simulink library "rect_model"  (R2018a)
settings: Solver=VariableStepAuto  StartTime=0.0  StopTime=10.0  RelTol=1e-3
libraries: powerlib x9
settings Model: Creator=ASUS  LastModifiedBy=ASUS

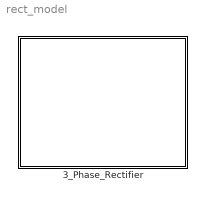
== system rect_model ==
  3_Phase_Rectifier : Subsystem

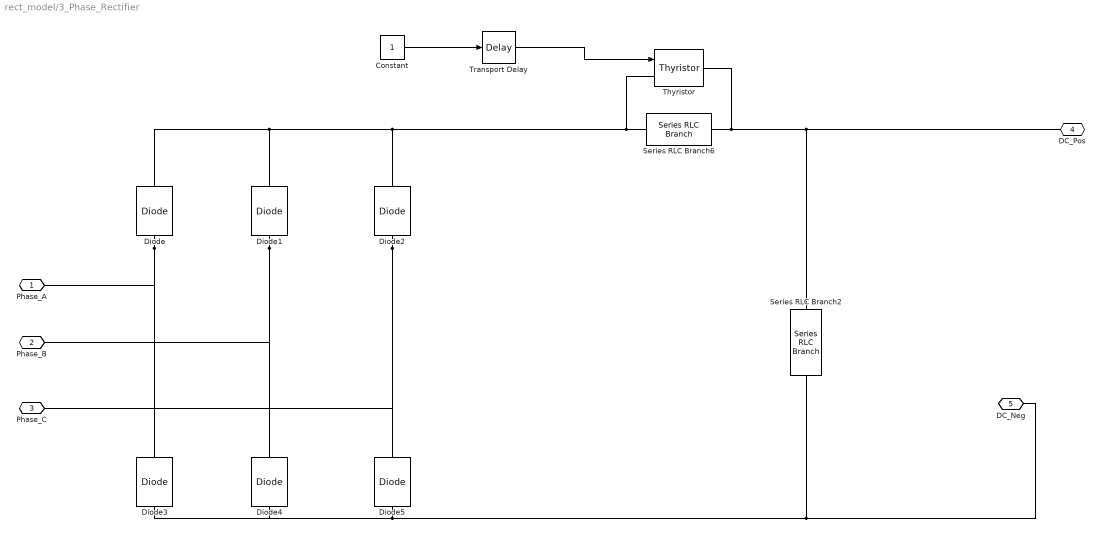
== system rect_model/3_Phase_Rectifier ==
  Constant : Constant
  Diode{,1..5} (6 alike) : powerlib/Power Electronics/Diode  Ron=0.001  Lon=0  Vf=0.8  IC=0  UseSnubber=0  Rs=500  Cs=250e-9  Measurements=off
  Series RLC Branch2 : powerlib/Elements/Series RLC Branch  LConnTagsString=__new0  RConnTagsString=__new0  BranchType=C  Resistance=72  Inductance=1e-3  SetiL0=off  InitialCurrent=0  Capacitance=2e-3  Setx0=off  InitialVoltage=0  Measurements=None
  Series RLC Branch6 : powerlib/Elements/Series RLC Branch  LConnTagsString=__new0  RConnTagsString=__new0  BranchType=R  Resistance=72  Inductance=1e-3  SetiL0=off  InitialCurrent=0  Capacitance=1e-6  Setx0=off  InitialVoltage=0  Measurements=None
  Thyristor : powerlib/Power Electronics/Thyristor  Ron=0.001  Lon=0  Vf=0.8  IC=0  Rs=500  Cs=250e-9  Measurements=off
  Transport Delay : TransportDelay  DelayTime=0.2
  Phase_A : PMIOPort  Side=Left
  Phase_B : PMIOPort  Port=2  Side=Left
  Phase_C : PMIOPort  Port=3  Side=Left
  DC_Pos : PMIOPort  Port=4  Side=Right
  DC_Neg : PMIOPort  Port=5  Side=Right
  wires:
  Transport Delay/1 -> Thyristor/1
  Constant/1 -> Transport Delay/1
  connections:
  Diode2/LConn1 -- Diode5/RConn1 -- Phase_C/RConn1
  Thyristor/LConn1 -- Series RLC Branch6/LConn1 -- Diode2/RConn1 -- Diode1/RConn1 -- Diode/RConn1
  Thyristor/RConn1 -- Series RLC Branch6/RConn1 -- Series RLC Branch2/LConn1 -- DC_Pos/RConn1
  Series RLC Branch2/RConn1 -- Diode3/LConn1 -- Diode4/LConn1 -- Diode5/LConn1 -- DC_Neg/RConn1
  Diode1/LConn1 -- Diode4/RConn1 -- Phase_B/RConn1
  Diode/LConn1 -- Diode3/RConn1 -- Phase_A/RConn1
